simulink model "Exemplu_figura7"  (R2016a)
settings: Solver=VariableStepDiscrete  StartTime=0.0  StopTime=30  RelTol=1e-3
undefined symbols (not defined in the file): entity, g, m, n
settings Model: Creator=Cristina  LastModifiedBy=Cristina

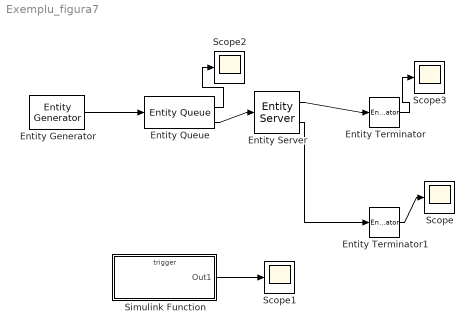
== system Exemplu_figura7 ==
  Entity Generator : EntityGenerator  OutputPortMessageModes=m  GenerateAction=|  ExitAction=g(entity.Priority);  AttributeName=Priority|ServiceTime  AttributeInitialValue=1|1.1  EntityType=Structured  EntityTypeName=Entity
      | if rand < 0.3
      |     entity.Priority = 1;
      | else
      |     entity.Priority = 2;
      | end
  Entity Queue : EntityQueue  InputPortMessageModes=m  OutputPortMessageModes=n,m  QueueType=Priority  PrioritySource=Priority  NumberEntitiesInBlock=on
      settings: OutputPortMap=o1,o5
  Entity Server : EntityServer  InputPortMessageModes=m  OutputPortMessageModes=m,m  Capacity=1  ServiceTimeValue=1.1  PermitPreemptionBasedOnAttribute=on  SortingAttributeName=Priority  WriteResidualTimeToAttribute=on  ResidualTimeAttributeName=ServiceTime
      settings: OutputPortMap=o9,o10
  Entity Terminator : EntityTerminator  InputPortMessageModes=m  NumberEntitiesArrived=on
      settings: OutputPortMap=o0
  Entity Terminator1 : EntityTerminator  InputPortMessageModes=m  NumberEntitiesArrived=on
      settings: OutputPortMap=o0
  Scope{,1..3} (4 alike) : Scope
  Simulink Function : Subsystem  TreatAsAtomicUnit=on
  wires:
  Entity Generator/1 -> Entity Queue/1
  Entity Queue/2 -> Entity Server/1
  Entity Server/1 -> Entity Terminator/1
  Entity Server/2 -> Entity Terminator1/1
  Entity Terminator1/1 -> Scope/1
  Simulink Function/1(Out1) -> Scope1/1
  Entity Queue/1 -> Scope2/1
  Entity Terminator/1 -> Scope3/1

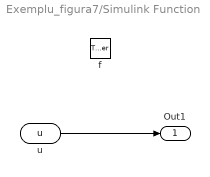
== system Exemplu_figura7/Simulink Function ==
  f : TriggerPort  TriggerType=function-call  IsSimulinkFunction=on  FunctionName=g  VariantControl=Variant
  u : ArgIn  DisableCoverage=on  ArgumentName=u
  Out1 : Outport
  wires:
  u/1 -> Out1/1
